simulink model "MODCTL"  (R2022b)
settings: configuration reference "SharedConfig" (kept outside this file)
values from neighbouring files (symbols this model uses):
  DrvModDialEna_C = 1.0    [MODCTL.sldd]
  DrvModDialVal_C : value not decoded    [MODCTL.sldd]
  DT_MODCTL_C = 0.1    [MODCTL.sldd]
  MotSpdReqThdModChg_C = 50.0    [MODCTL.sldd]
  MotSpdThdModChg_C = 50.0    [MODCTL.sldd]
  MotTqReqThdModChg_C = 1.0    [MODCTL.sldd]
  PwrCmdDialEna_C = 1.0    [MODCTL.sldd]
  PwrCmdDialVal_C = 0.0    [MODCTL.sldd]
  WakeRetry_C = 0.0    [MODCTL.sldd]
  WakeTout_C = 1.0    [MODCTL.sldd]
undefined symbols (not defined in the file or in its folder): slcm
libraries: simulink x1
Description:
  | Determines the operating mode of the drive inverter.
settings Model: DataDictionary=MODCTL.sldd  Creator=Kevin  LastModifiedBy=Max Kolesnikov
settings ConfigSetRef: SourceName=SharedConfig

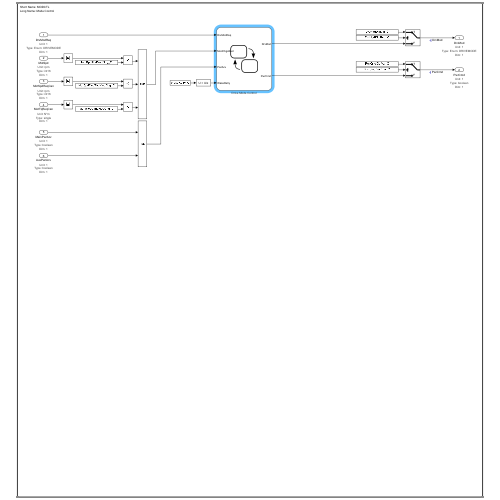
[thumbnail: Simulink's stored preview of the top-level diagram]
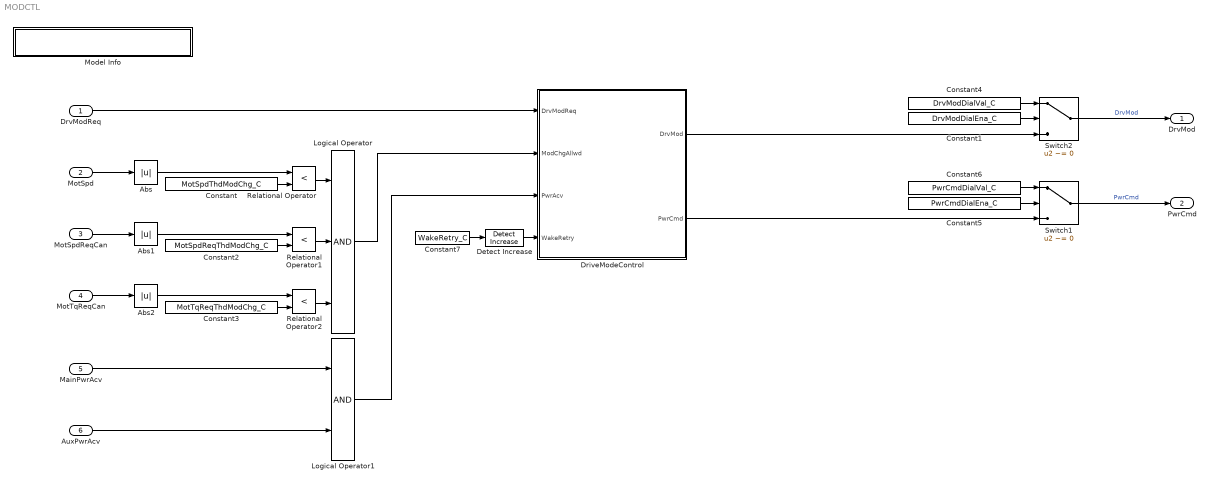
== system MODCTL ==
  DrvModReq : Inport  OutDataTypeStr=Enum: DRIVEMODE  Unit=1  PortDimensions=1
      settings: AttributesFormatString=|
      | Unit: %<Unit>
      | Type: %<OutDataTypeStr>
      | Dim: %<PortDimensions>
  MotSpd : Inport  Port=2  OutDataTypeStr=int16  Unit=rpm  PortDimensions=1
      settings: AttributesFormatString=|
      | Unit: %<Unit>
      | Type: %<OutDataTypeStr>
      | Dim: %<PortDimensions>
  MotSpdReqCan : Inport  Port=3  OutDataTypeStr=int16  Unit=rpm  PortDimensions=1
      settings: AttributesFormatString=|
      | Unit: %<Unit>
      | Type: %<OutDataTypeStr>
      | Dim: %<PortDimensions>
  MotTqReqCan : Inport  Port=4  OutDataTypeStr=single  Unit=N*m  PortDimensions=1
      settings: AttributesFormatString=|
      | Unit: %<Unit>
      | Type: %<OutDataTypeStr>
      | Dim: %<PortDimensions>
  MainPwrAcv : Inport  Port=5  OutDataTypeStr=boolean  Unit=1  PortDimensions=1
      settings: AttributesFormatString=|
      | Unit: %<Unit>
      | Type: %<OutDataTypeStr>
      | Dim: %<PortDimensions>
  AuxPwrAcv : Inport  Port=6  OutDataTypeStr=boolean  Unit=1  PortDimensions=1
      settings: AttributesFormatString=|
      | Unit: %<Unit>
      | Type: %<OutDataTypeStr>
      | Dim: %<PortDimensions>
  Abs : Abs  SaturateOnIntegerOverflow=off
  Abs1 : Abs  SaturateOnIntegerOverflow=off
  Abs2 : Abs  SaturateOnIntegerOverflow=off
  Constant : Constant  Value=MotSpdThdModChg_C
  Constant1 : Constant  Value=DrvModDialEna_C
  Constant2 : Constant  Value=MotSpdReqThdModChg_C
  Constant3 : Constant  Value=MotTqReqThdModChg_C
  Constant4 : Constant  Value=DrvModDialVal_C
  Constant5 : Constant  Value=PwrCmdDialEna_C
  Constant6 : Constant  Value=PwrCmdDialVal_C
  Constant7 : Constant  Value=WakeRetry_C
  Detect Increase : simulink/Logic and Bit Operations/Detect Increase  vinit=0.0  OutDataTypeStr=boolean
  DriveModeControl : Stateflow chart  Description=Drive Mode Control  TreatAsAtomicUnit=on
      settings: AttributesFormatString=%<Description>
  Logical Operator : Logic  Inputs=3  AllPortsSameDT=off  OutDataTypeStr=boolean
  Logical Operator1 : Logic  AllPortsSameDT=off  OutDataTypeStr=boolean
  Model Info : Subsystem  LoadFcn=slcm LoadBlock;  InitFcn=slcm('UpdateAllCMBlocksInThisModelInit')  mask(CMBlock){Frame=off, DisplayStringWithTags=|, MaskDisplayString=Short Name: MODCTL\nLong Name: Mode Control, HorizontalTextAlignment=Left, LeftAlignmentValue=0.02}
      mask DisplayStringWithTags=|
      | Short Name: %<ModelName>
      | Long Name: Mode Control
      mask prompts: Frame "Simulink:masks:Frame_MP"; DisplayStringWithTags "Simulink:masks:DisplayStringWithTags_MP"; MaskDisplayString "Simulink:masks:MaskDisplayString_MP"; HorizontalTextAlignment "Simulink:masks:HorizontalTextAlignment_MP"; LeftAlignmentValue "Simulink:masks:LeftAlignmentValue_MP"
      mask help: Simulink:masks:CMBlock_MD
      settings: CopyFcn=slcm CopyBlock;  DeleteFcn=slcm Cancel;  PostSaveFcn=slcm('UpdateAllCMBlocksInThisModel')  NameChangeFcn=slcm Rename;  OpenFcn=slcm
      mask Display: text(slResolve(LeftAlignmentValue, gcbh), 0.5, MaskDisplayString, 'HorizontalAlignment', HorizontalTextAlignment)
  Relational Operator : RelationalOperator  Operator=<  OutDataTypeStr=boolean  RndMeth=Simplest  InputSameDT=off
  Relational Operator1 : RelationalOperator  Operator=<  OutDataTypeStr=boolean  RndMeth=Simplest  InputSameDT=off
  Relational Operator2 : RelationalOperator  Operator=<  OutDataTypeStr=boolean  RndMeth=Simplest  InputSameDT=off
  Switch1 : Switch  Criteria=u2 ~= 0  SaturateOnIntegerOverflow=off  InputSameDT=off
  Switch2 : Switch  Criteria=u2 ~= 0  SaturateOnIntegerOverflow=off  InputSameDT=off
  DrvMod : Outport  OutDataTypeStr=Enum: DRIVEMODE  Unit=1  PortDimensions=1
      settings: AttributesFormatString=|
      | Unit: %<Unit>
      | Type: %<OutDataTypeStr>
      | Dim: %<PortDimensions>
  PwrCmd : Outport  Port=2  OutDataTypeStr=boolean  Unit=1  PortDimensions=1
      settings: AttributesFormatString=|
      | Unit: %<Unit>
      | Type: %<OutDataTypeStr>
      | Dim: %<PortDimensions>
  wires:
  Switch2/1 -> DrvMod/1  "DrvMod"
  Constant1/1 -> Switch2/2
  Constant4/1 -> Switch2/1
  DriveModeControl/1(DrvMod) -> Switch2/3
  MotSpd/1 -> Abs/1
  MotSpdReqCan/1 -> Abs1/1
  MotTqReqCan/1 -> Abs2/1
  Abs/1 -> Relational Operator/1
  Abs1/1 -> Relational Operator1/1
  Abs2/1 -> Relational Operator2/1
  Constant/1 -> Relational Operator/2
  Constant2/1 -> Relational Operator1/2
  Constant3/1 -> Relational Operator2/2
  Relational Operator1/1 -> Logical Operator/2
  Relational Operator/1 -> Logical Operator/1
  Relational Operator2/1 -> Logical Operator/3
  DrvModReq/1 -> DriveModeControl/1(DrvModReq)
  Logical Operator/1 -> DriveModeControl/2(ModChgAllwd)
  MainPwrAcv/1 -> Logical Operator1/1
  AuxPwrAcv/1 -> Logical Operator1/2
  Logical Operator1/1 -> DriveModeControl/3(PwrAcv)
  Constant6/1 -> Switch1/1
  Constant5/1 -> Switch1/2
  Switch1/1 -> PwrCmd/1  "PwrCmd"
  DriveModeControl/2(PwrCmd) -> Switch1/3
  Detect Increase/1 -> DriveModeControl/4(WakeRetry)
  Constant7/1 -> Detect Increase/1

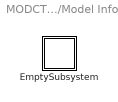
== system MODCTL/Model Info ==
  EmptySubsystem : Subsystem

== system MODCTL/Model Info/EmptySubsystem ==

== stateflow chart MODCTL/DriveModeControl ==
  state WAKE
    en:
    Tmr = 0;
    du:
    DrvMod = DISABLED;
    PwrCmd = true;
    Tmr = Tmr + DT_MODCTL_C;
  state POWER_ERROR
    du:
    DrvMod = DISABLED;
    PwrCmd = false;
  state ACTIVE
    du:
    PwrCmd = true;
    state DISABLED
      DrvMod = DISABLED;
    state OPEN_LOOP
      DrvMod = OPEN_LOOP;
    state TORQUE
      DrvMod = TQ_CTRL;
    state SPEED
      DrvMod = SPD_CTRL;
    (default) -> DISABLED
    (junction 50) -> (junction 57)
    (junction 57) -> DISABLED
    DISABLED -> (junction 37) : [DrvModReq ~= DISABLED && ...
        | ModChgAllwd]
    (junction 54) -> (junction 50)
    (junction 64) -> (junction 57) [order 2]
    (junction 37) -> (junction 29)
    (junction 64) -> OPEN_LOOP [order 1] : [DrvModReq == OPEN_LOOP]
    OPEN_LOOP -> (junction 29) : [DrvModReq ~= OPEN_LOOP]
    (junction 46) -> (junction 64) [order 2]
    (junction 29) -> (junction 31)
    (junction 46) -> TORQUE [order 1] : [DrvModReq == TQ_CTRL]
    TORQUE -> (junction 31) : [DrvModReq ~= TQ_CTRL]
    (junction 44) -> (junction 46) [order 2]
    (junction 31) -> (junction 33)
    (junction 44) -> SPEED [order 1] : [DrvModReq == SPD_CTRL]
    SPEED -> (junction 33) : [DrvModReq ~= SPD_CTRL]
    (junction 60) -> (junction 44) [order 1] : [ModChgAllwd]
    (junction 33) -> (junction 52)
    (junction 60) -> (junction 54) [order 2]
    (junction 52) -> (junction 60)
  (default) -> WAKE
  POWER_ERROR -> WAKE : [WakeRetry]
  WAKE -> POWER_ERROR [order 1] : [Tmr >= WakeTout_C]
  WAKE -> ACTIVE [order 2] : [PwrAcv]
  ACTIVE -> POWER_ERROR : [~PwrAcv]
  data: DrvModReq input; DrvMod output Enum: DRIVEMODE; ModChgAllwd input; PwrCmd output boolean; PwrAcv input; WakeRetry input; WakeTout_C parameter; Tmr local single; DT_MODCTL_C parameter
